simulink model "SimulinkScope"  (Simulink 7.6)
settings: Solver=ode45  StartTime=0.0  StopTime=10.0  RelTol=1e-3
undefined symbols (not defined in the file or in its folder): mu
settings Model: Creator=Administrator  LastModifiedBy=Administrator

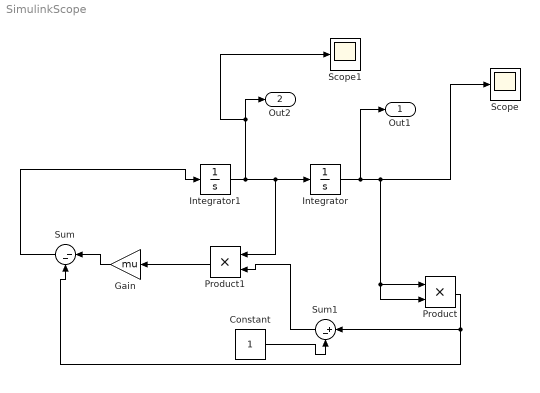
== system SimulinkScope ==
  Constant : Constant
  Gain : Gain  Gain=mu
  Integrator : Integrator  InitialCondition=2
  Integrator1 : Integrator  InitialCondition=-2
  Product : Product  RndMeth=Zero
  Product1 : Product  RndMeth=Zero
  Scope : Scope
  Scope1 : Scope
  Sum : Sum  Inputs=|--
  Sum1 : Sum  Inputs=|+-
  Out1 : Outport
  Out2 : Outport  Port=2
  wires:
  Integrator1/1 -> Integrator/1, Product1/1, Out2/1, Scope1/1
  Integrator/1 -> Out1/1, Product/1, Product/2, Scope/1
  Product/1 -> Sum/2, Sum1/1
  Constant/1 -> Sum1/2
  Sum1/1 -> Product1/2
  Product1/1 -> Gain/1
  Gain/1 -> Sum/1
  Sum/1 -> Integrator1/1
